simulink model "ex_long_lat_dynamics_charcrit_speed"  (R2026a)
settings: Solver=VariableStepAuto  StopTime=10
libraries: aerolibconvert2 x2, simulink x1
settings Model: Creator=doyeop  LastModifiedBy=doyeop

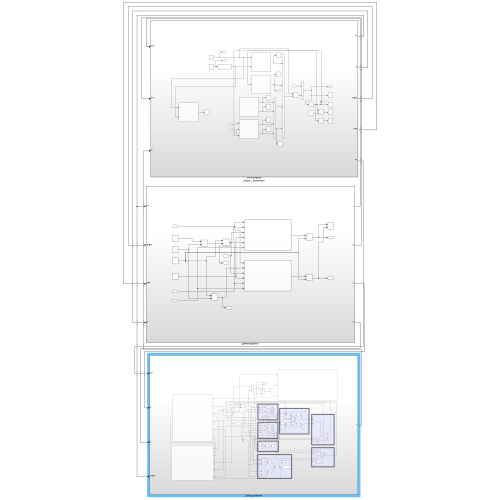
[thumbnail: Simulink's stored preview of the top-level diagram]
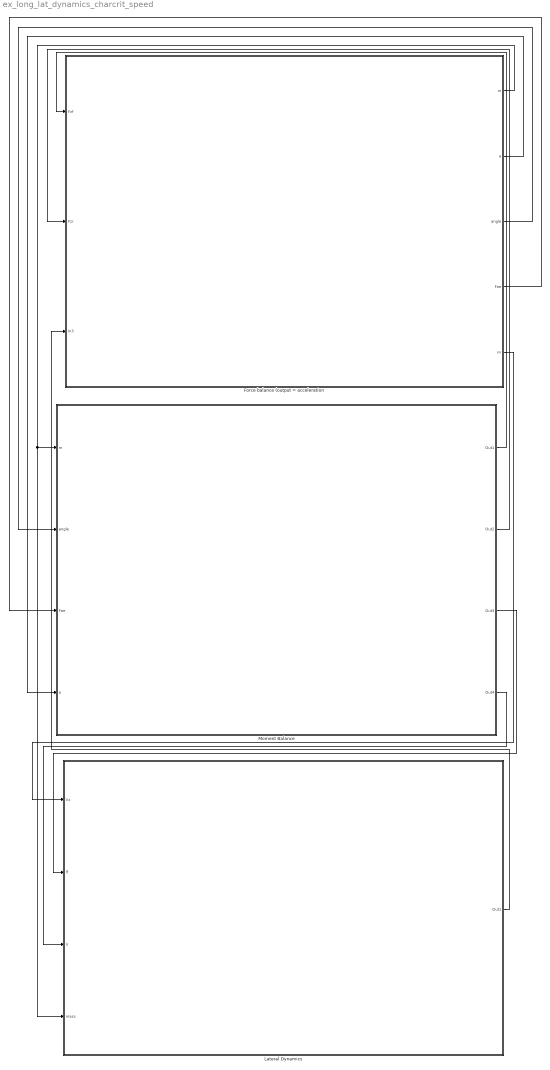
== system ex_long_lat_dynamics_charcrit_speed ==
  Force balance (output = acceleration : Subsystem
  Lateral Dynamics : Subsystem
  Moment Balance : Subsystem
  wires:
  Force balance (output = acceleration/1(m) -> Lateral Dynamics/4(mass), Moment Balance/1(m)
  Force balance (output = acceleration/2(a) -> Moment Balance/4(a)
  Force balance (output = acceleration/3(angle) -> Moment Balance/2(angle)
  Force balance (output = acceleration/4(Fae) -> Moment Balance/3(Fae)
  Moment Balance/1(Out1) -> Force balance (output = acceleration/1(Fzf)
  Moment Balance/2(Out2) -> Force balance (output = acceleration/2(Fzr)
  Force balance (output = acceleration/5(vx) -> Lateral Dynamics/1(Vx)
  Moment Balance/3(Out3) -> Lateral Dynamics/2(lf)
  Moment Balance/4(Out4) -> Lateral Dynamics/3(lr)
  Lateral Dynamics/1(Out1) -> Force balance (output = acceleration/3(In3)

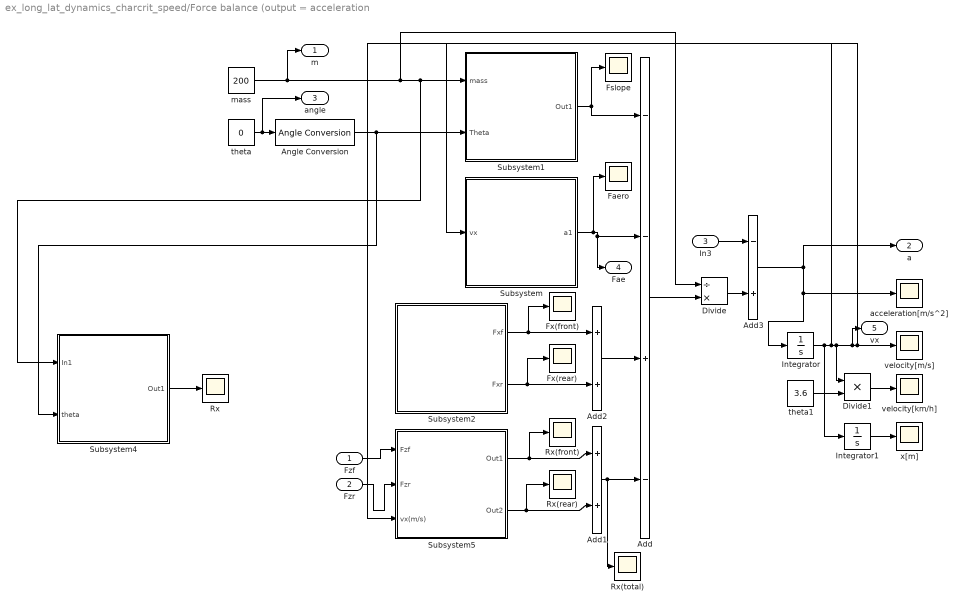
== system ex_long_lat_dynamics_charcrit_speed/Force balance (output = acceleration ==
  Fzf : Inport
  Fzr : Inport  Port=2
  In3 : Inport  Port=3
  Add : Sum  Inputs=--+-
  Add1 : Sum
  Add2 : Sum
  Add3 : Sum  Inputs=-+
  Angle Conversion : aerolibconvert2/Angle Conversion  IU=deg  OU=rad
  Divide : Product  Inputs=/*
  Divide1 : Product  Inputs=**
  Faero : Scope
      settings: ActiveDisplayYMinimum=-21.806973838724872  ActiveDisplayYMaximum=245.93181269445461  DataLoggingVariableName=ScopeData4
  Fslope : Scope
      settings: ActiveDisplayYMinimum=467.68768501992645  ActiveDisplayYMaximum=4126.826484026702  DataLoggingVariableName=ScopeData3
  Fx(front) : Scope
      settings: ActiveDisplayYMinimum=-0.77322383064043154  ActiveDisplayYMaximum=0.91988628090500946  DataLoggingVariableName=ScopeData5
  Fx(rear) : Scope
      settings: ActiveDisplayYMinimum=-0.77322383064043154  ActiveDisplayYMaximum=0.91988628090500946  DataLoggingVariableName=ScopeData10
  Integrator : Integrator
  Integrator1 : Integrator
  Rx : Scope
      settings: ActiveDisplayYMinimum=21.392000000000003  ActiveDisplayYMaximum=41.392  DataLoggingVariableName=ScopeData6
  Rx(front) : Scope
      settings: ActiveDisplayYMinimum=-1  ActiveDisplayYMaximum=1  DataLoggingVariableName=ScopeData11
  Rx(rear) : Scope
      settings: ActiveDisplayYMinimum=-1  ActiveDisplayYMaximum=1  DataLoggingVariableName=ScopeData12
  Rx(total) : Scope
      settings: ActiveDisplayYMinimum=26.459225679325527  ActiveDisplayYMaximum=38.083177364358953  DataLoggingVariableName=ScopeData13
  Subsystem : Subsystem
  Subsystem1 : Subsystem
  Subsystem2 : Subsystem
  Subsystem4 : Subsystem
  Subsystem5 : Subsystem
  acceleration[m/s^2] : Scope
      settings: ActiveDisplayYMinimum=-1  ActiveDisplayYMaximum=1
  mass : Constant  Value=200  SampleTime=-1
  theta : Constant  Value=0  SampleTime=-1
  theta1 : Constant  Value=3.6  SampleTime=-1
  velocity[km/h] : Scope
      settings: ActiveDisplayYMinimum=-12.890564976943338  ActiveDisplayYMaximum=101.85529757372632  DataLoggingVariableName=ScopeData7
  velocity[m/s] : Scope
      settings: ActiveDisplayYMinimum=-1  ActiveDisplayYMaximum=1
  x[m] : Scope
      settings: ActiveDisplayYMinimum=-1  ActiveDisplayYMaximum=1  DataLoggingVariableName=ScopeData2
  m : Outport
  a : Outport  Port=2
  angle : Outport  Port=3
  Fae : Outport  Port=4
  vx : Outport  Port=5
  wires:
  Divide1/1 -> velocity[km/h]/1
  Subsystem/1(a1) -> Faero/1, Add/2, Fae/1
  Integrator1/1 -> x[m]/1
  Add/1 -> Divide/2
  Angle Conversion/1 -> Subsystem4/2(theta), Subsystem1/2(Theta)
  Divide/1 -> Add3/2
  mass/1 -> m/1, Divide/1, Subsystem4/1(In1), Subsystem1/1(mass)
  Subsystem2/1(Fxf) -> Add2/1, Fx(front)/1
  theta1/1 -> Divide1/2
  Integrator/1 -> Integrator1/1, Subsystem/1(vx), Divide1/1, vx/1, Subsystem5/3(vx(m/s)), velocity[m/s]/1
  Subsystem1/1(Out1) -> Fslope/1, Add/1
  Subsystem4/1(Out1) -> Rx/1
  theta/1 -> angle/1, Angle Conversion/1
  Subsystem2/2(Fxr) -> Fx(rear)/1, Add2/2
  Fzf/1 -> Subsystem5/1(Fzf)
  Fzr/1 -> Subsystem5/2(Fzr)
  Add1/1 -> Add/4, Rx(total)/1
  Subsystem5/2(Out2) -> Rx(rear)/1, Add1/2
  Subsystem5/1(Out1) -> Rx(front)/1, Add1/1
  Add2/1 -> Add/3
  In3/1 -> Add3/1
  Add3/1 -> Integrator/1, acceleration[m/s^2]/1, a/1

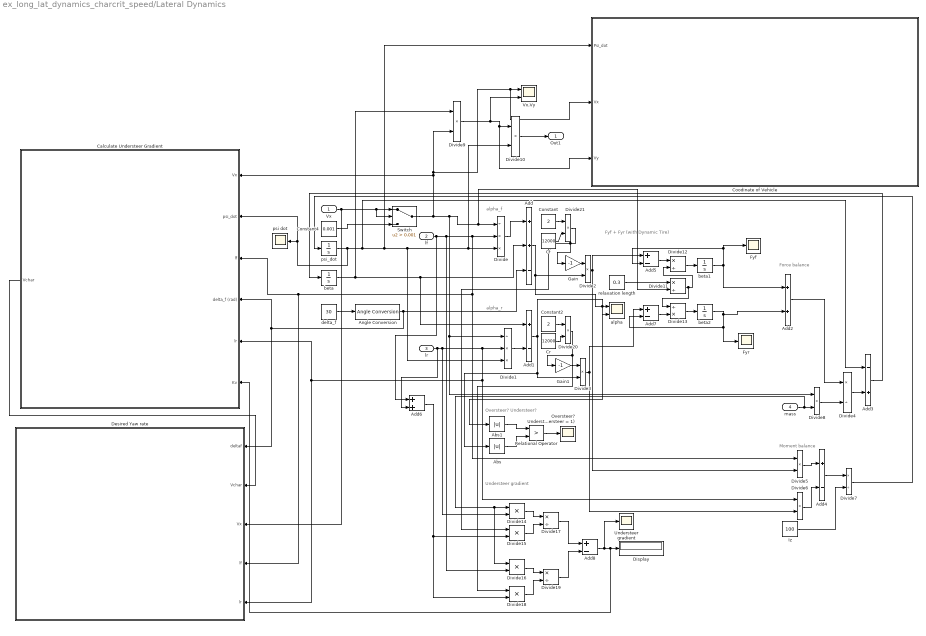
== system ex_long_lat_dynamics_charcrit_speed/Lateral Dynamics ==
  note: Understeer gradient
  note: Oversteer? Understeer?
  note: Moment balance
  note: Force balance
  note: Fyf + Fyr (with Dynamic Tire)
  note: alpha_r
  note: alpha_f
  Vx : Inport
  lf : Inport  Port=2
  lr : Inport  Port=3
  mass : Inport  Port=4
  Abs : Abs  SaturateOnIntegerOverflow=off
  Abs1 : Abs  SaturateOnIntegerOverflow=off
  Add : Sum  Inputs=++-
  Add{1,4..5,7..8} (5 alike) : Sum  Inputs=+-
  Add2 : Sum
  Add3 : Sum  Inputs=-+
  Add6 : Sum
  Angle Conversion : aerolibconvert2/Angle Conversion  IU=deg  OU=rad
  Calculate Understeer Gradient : Subsystem
  Cf : Constant  Value=12000  SampleTime=-1
  Constant : Constant  Value=2  SampleTime=-1
  Constant2 : Constant  Value=2  SampleTime=-1
  Constant4 : Constant  Value=0.001
  Coodinate of Vehicle : Subsystem
  Cr : Constant  Value=12000  SampleTime=-1
  Desired Yaw rate : Subsystem
  Display : Display
  Divide : Product  Inputs=/**
  Divide1 : Product  Inputs=/**
  Divide{5..6,8..10,14..16,18} (9 alike) : Product  Inputs=**
  Divide{4,7,11..12,17,19} (6 alike) : Product  Inputs=*/
  Divide13 : Product  Inputs=/*
  Divide{2..3,20..21} (4 alike) : Product
  Fyf : Scope
      settings: ActiveDisplayYMinimum=-170.39599626491659  ActiveDisplayYMaximum=1134.9817554046469  DataLoggingVariableName=ScopeData14
  Fyr : Scope
      settings: ActiveDisplayYMinimum=-197.89133133597571  ActiveDisplayYMaximum=765.23113635108643  DataLoggingVariableName=ScopeData15
  Gain : Gain  Gain=-1
  Gain1 : Gain  Gain=-1
  Iz : Constant  Value=100  SampleTime=-1
  Oversteer? Understeer? (Understeer = 1) : Scope
      settings: ActiveDisplayYMinimum=-0.12499999999999997  ActiveDisplayYMaximum=1.125  DataLoggingVariableName=ScopeData28
  Relational Operator : RelationalOperator  Operator=>  OutDataTypeStr=boolean  RndMeth=Simplest  InputSameDT=off
  Switch : Switch  Criteria=u2 > Threshold  Threshold=0.001  SaturateOnIntegerOverflow=off  InputSameDT=off
  Understeer gradient : Scope
      settings: ActiveDisplayYMinimum=0.0006666666666666661  ActiveDisplayYMaximum=0.0026666666666666661  DataLoggingVariableName=ScopeData9
  Vx,Vy : Scope  NumInputPorts=2
      settings: ActiveDisplayYMinimum=-0.84716123690803014  ActiveDisplayYMaximum=7.6244511321722737  DataLoggingVariableName=ScopeData16
  alpha : Scope  NumInputPorts=2
      settings: ActiveDisplayYMinimum=-0.10159314992994704  ActiveDisplayYMaximum=0.04167372337235864  DataLoggingVariableName=ScopeData27
  beta : Integrator
  beta1 : Integrator
  beta2 : Integrator
  delta_f : Constant  Value=30  SampleTime=-1
  psi dot : Scope
      settings: ActiveDisplayYMinimum=-0.20399598787459142  ActiveDisplayYMaximum=1.8359638908713232  DataLoggingVariableName=ScopeData17
  psi_dot : Integrator
  relaxation length : Constant  Value=0.3
  Out1 : Outport
  wires:
  beta/1 -> Divide9/1, Add1/1, Add/2
  Divide/1 -> Add/1
  lr/1 -> Add6/2, Divide14/2, Divide6/1, Desired Yaw rate/5(lr), Calculate Understeer Gradient/5(lr), Divide1/2
  Divide1/1 -> Add1/2
  Add/1 -> Abs1/1, alpha/1, Divide2/2
  Cf/1 -> Divide21/2
  Add1/1 -> Abs/1, Divide3/2, alpha/2
  Cr/1 -> Divide20/2
  Divide2/1 -> Add5/1, Divide5/2
  Divide3/1 -> Add7/1, Divide6/2
  Divide4/1 -> Add3/2
  Add3/1 -> beta/1
  lf/1 -> Divide16/2, Divide5/1, Desired Yaw rate/4(lf), Calculate Understeer Gradient/3(lf), Divide/2, Add6/1
  Divide5/1 -> Add4/1
  Divide6/1 -> Add4/2
  Add4/1 -> Divide7/1
  Iz/1 -> Divide7/2
  Divide7/1 -> psi_dot/1
  Vx/1 -> Switch/2, Switch/1, Desired Yaw rate/3(Vx)
  Constant4/1 -> Switch/3
  mass/1 -> Divide14/1, Divide16/1, Divide8/2
  Divide8/1 -> Divide4/2
  Add2/1 -> Divide4/1
  delta_f/1 -> Angle Conversion/1
  beta1/1 -> Fyf/1, Add5/2, Add2/1
  beta2/1 -> Add7/2, Fyr/1, Add2/2
  Abs1/1 -> Relational Operator/1
  Abs/1 -> Relational Operator/2
  Relational Operator/1 -> Oversteer? Understeer? (Understeer = 1)/1
  Divide9/1 -> Coodinate of Vehicle/3(Vy), Divide10/1, Vx,Vy/2
  Divide10/1 -> Out1/1
  Switch/1 -> Divide8/1, Divide1/1, Divide11/2, Divide/1, Divide9/2, Coodinate of Vehicle/2(Vx), Vx,Vy/1, Calculate Understeer Gradient/1(Vx)
  Divide12/1 -> beta1/1
  Add5/1 -> Divide12/1
  Divide11/1 -> Divide13/1, Divide12/2
  Add7/1 -> Divide13/2
  Divide13/1 -> beta2/1
  relaxation length/1 -> Divide11/1
  Add6/1 -> Divide18/2, Divide15/2
  Divide14/1 -> Divide17/1
  Divide15/1 -> Divide17/2
  Divide16/1 -> Divide19/1
  Divide18/1 -> Divide19/2
  Divide19/1 -> Add8/2
  Divide17/1 -> Add8/1
  Add8/1 -> Calculate Understeer Gradient/6(Kv), Display/1, Understeer gradient/1
  Angle Conversion/1 -> Add/3, Desired Yaw rate/1(deltaf), Calculate Understeer Gradient/4(delta_f (rad))
  psi_dot/1 -> psi dot/1, Calculate Understeer Gradient/2(psi_dot), Add3/1, Coodinate of Vehicle/1(Psi_dot), Divide/3, Divide10/2, Divide1/3
  Constant2/1 -> Divide20/1
  Divide20/1 -> Gain1/1, Divide18/1
  Constant/1 -> Divide21/1
  Divide21/1 -> Divide15/1, Gain/1
  Gain/1 -> Divide2/1
  Gain1/1 -> Divide3/1
  Calculate Understeer Gradient/1(Vchar) -> Desired Yaw rate/2(Vchar)

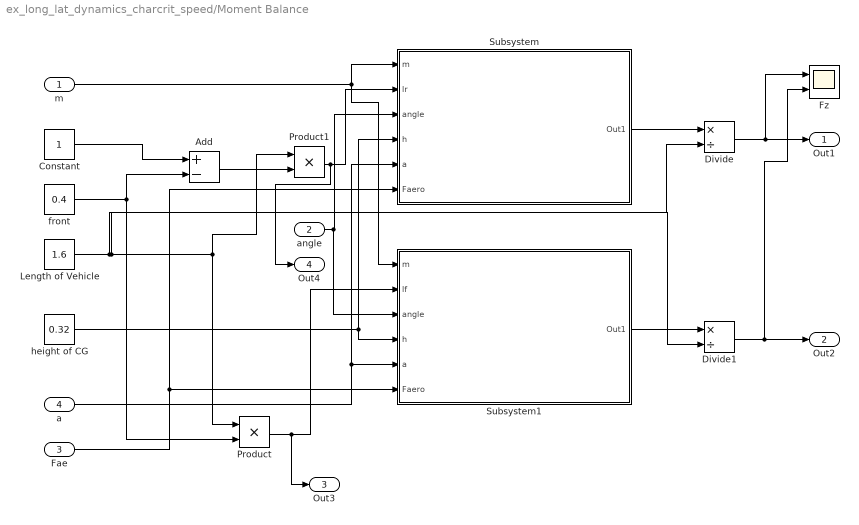
== system ex_long_lat_dynamics_charcrit_speed/Moment Balance ==
  m : Inport
  angle : Inport  Port=2
  Fae : Inport  Port=3
  a : Inport  Port=4
  Add : Sum  Inputs=+-
  Constant : Constant
  Divide : Product  Inputs=*/
  Divide1 : Product  Inputs=*/
  Fz : Scope  NumInputPorts=2
      settings: ActiveDisplayYMinimum=618.58251067683113  ActiveDisplayYMaximum=1343.5454915820123  DataLoggingVariableName=ScopeData8
  Length of Vehicle : Constant  Value=1.6  SampleTime=-1
  Product : Product
  Product1 : Product
  Subsystem : Subsystem
  Subsystem1 : Subsystem
  front : Constant  Value=0.4  SampleTime=-1
  height of CG : Constant  Value=0.32
  Out1 : Outport
  Out2 : Outport  Port=2
  Out3 : Outport  Port=3
  Out4 : Outport  Port=4
  wires:
  m/1 -> Subsystem1/1(m), Subsystem/1(m)
  angle/1 -> Subsystem1/3(angle), Subsystem/3(angle)
  front/1 -> Product/2, Add/2
  Constant/1 -> Add/1
  Length of Vehicle/1 -> Divide/2, Divide1/2, Product1/1, Product/1
  Add/1 -> Product1/2
  Product1/1 -> Out4/1, Subsystem/2(lr)
  height of CG/1 -> Subsystem/4(h), Subsystem1/4(h)
  a/1 -> Subsystem1/5(a), Subsystem/5(a)
  Fae/1 -> Subsystem1/6(Faero), Subsystem/6(Faero)
  Subsystem/1(Out1) -> Divide/1
  Subsystem1/1(Out1) -> Divide1/1
  Product/1 -> Out3/1, Subsystem1/2(lf)
  Divide/1 -> Out1/1, Fz/1
  Divide1/1 -> Fz/2, Out2/1

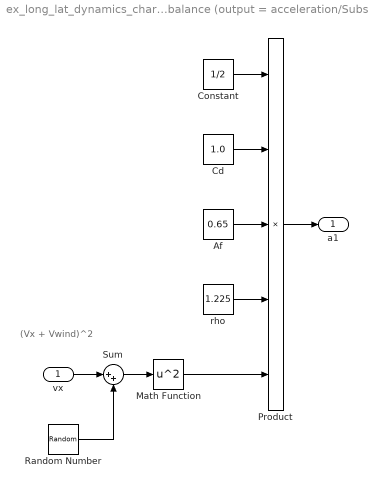
== system ex_long_lat_dynamics_charcrit_speed/Force balance (output = acceleration/Subsystem ==
  note: (Vx + Vwind)^2
  vx : Inport
  Af : Constant  Value=0.65  SampleTime=-1
  Cd : Constant  Value=1.0  SampleTime=-1
  Constant : Constant  Value=1/2  SampleTime=-1
  Math Function : Math  Operator=square
  Product : Product  Inputs=5
  Random Number : RandomNumber  Mean=3  Variance=0.5^2  SampleTime=0.1
  Sum : Sum  Inputs=|++
  rho : Constant  Value=1.225  SampleTime=-1
  a1 : Outport
  wires:
  Cd/1 -> Product/2
  Af/1 -> Product/3
  Constant/1 -> Product/1
  rho/1 -> Product/4
  Random Number/1 -> Sum/2
  vx/1 -> Sum/1
  Sum/1 -> Math Function/1
  Math Function/1 -> Product/5
  Product/1 -> a1/1

== system ex_long_lat_dynamics_charcrit_speed/Force balance (output = acceleration/Subsystem1 ==
  mass : Inport
  Theta : Inport  Port=2
  Constant : Constant  Value=9.81  SampleTime=-1
  Product : Product  Inputs=3
  Trigonometric Function : Trigonometry
  Out1 : Outport
  wires:
  mass/1 -> Product/1
  Theta/1 -> Trigonometric Function/1
  Trigonometric Function/1 -> Product/3
  Constant/1 -> Product/2
  Product/1 -> Out1/1

== system ex_long_lat_dynamics_charcrit_speed/Force balance (output = acceleration/Subsystem2 ==
  Constant : Constant  Value=0  SampleTime=-1
  Constant1 : Constant  Value=500  SampleTime=-1
  Fxf : Outport
  Fxr : Outport  Port=2
  wires:
  Constant/1 -> Fxf/1
  Constant1/1 -> Fxr/1

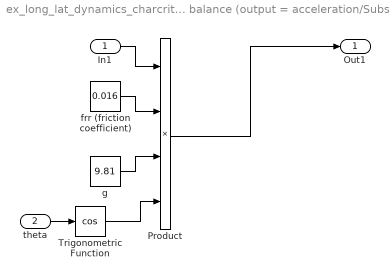
== system ex_long_lat_dynamics_charcrit_speed/Force balance (output = acceleration/Subsystem4 ==
  In1 : Inport
  theta : Inport  Port=2
  Product : Product  Inputs=4
  Trigonometric Function : Trigonometry  Operator=cos
  frr (friction coefficient) : Constant  Value=0.016  SampleTime=-1
  g : Constant  Value=9.81  SampleTime=-1
  Out1 : Outport
  wires:
  In1/1 -> Product/1
  frr (friction coefficient)/1 -> Product/2
  g/1 -> Product/3
  theta/1 -> Trigonometric Function/1
  Product/1 -> Out1/1
  Trigonometric Function/1 -> Product/4

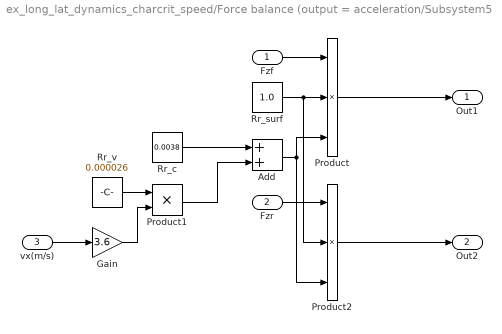
== system ex_long_lat_dynamics_charcrit_speed/Force balance (output = acceleration/Subsystem5 ==
  Fzf : Inport
  Fzr : Inport  Port=2
  vx(m/s) : Inport  Port=3
  Add : Sum
  Gain : Gain  Gain=3.6
  Product : Product  Inputs=3
  Product1 : Product
  Product2 : Product  Inputs=3
  Rr_c : Constant  Value=0.0038  SampleTime=-1
  Rr_surf : Constant  Value=1.0  SampleTime=-1
  Rr_v : Constant  Value=0.000026  SampleTime=-1
  Out1 : Outport
  Out2 : Outport  Port=2
  wires:
  Fzf/1 -> Product/1
  Product/1 -> Out1/1
  Rr_surf/1 -> Product2/2, Product/2
  Rr_v/1 -> Product1/1
  vx(m/s)/1 -> Gain/1
  Product1/1 -> Add/2
  Rr_c/1 -> Add/1
  Add/1 -> Product2/3, Product/3
  Gain/1 -> Product1/2
  Fzr/1 -> Product2/1
  Product2/1 -> Out2/1

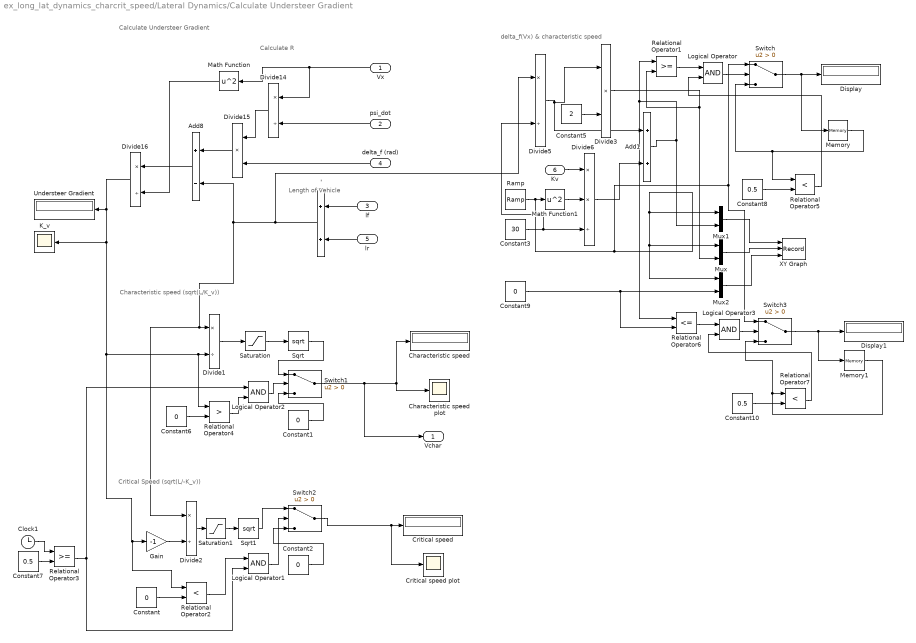
== system ex_long_lat_dynamics_charcrit_speed/Lateral Dynamics/Calculate Understeer Gradient ==
  note: delta_f(Vx) & characteristic speed
  note: Critical Speed
      | (sqrt(L/-K_v))
  note: Characteristic speed
      | (sqrt(L/K_v))
  note: Length of Vehicle
  note: Calculate Understeer Gradient
  note: Calculate R
  Vx : Inport
  psi_dot : Inport  Port=2
  lf : Inport  Port=3
  delta_f (rad) : Inport  Port=4
  lr : Inport  Port=5
  Kv : Inport  Port=6
  ' : Sum
  Add1 : Sum
  Add8 : Sum  Inputs=+-
  Characteristic speed : Display
  Characteristic speed plot : Scope
      settings: ActiveDisplayYMinimum=-3.8779477371123048  ActiveDisplayYMaximum=34.90152963401075  DataLoggingVariableName=ScopeData19
  Clock1 : Clock
  Constant{,1..2,6} (4 alike) : Constant  Value=0
  Constant10 : Constant  Value=0.5
  Constant3 : Constant  Value=30
  Constant5 : Constant  Value=2
  Constant7 : Constant  Value=0.5  SampleTime=-1
  Constant8 : Constant  Value=0.5
  Constant9 : Constant  Value=0  SampleTime=-1
  Critical speed : Display
  Critical speed plot : Scope
      settings: ActiveDisplayYMinimum=-4.4232312925042283  ActiveDisplayYMaximum=39.80908163253806  DataLoggingVariableName=ScopeData21
  Display : Display
  Display1 : Display
  Divide{1..2,5,14,16} (5 alike) : Product  Inputs=*/
  Divide15 : Product  Inputs=**
  Divide3 : Product  Inputs=**
  Divide6 : Product  Inputs=**/
  Gain : Gain  Gain=-1
  K_v : Scope
      settings: ActiveDisplayYMinimum=-33.664212716268274  ActiveDisplayYMaximum=291.42077077577937  DataLoggingVariableName=ScopeData18
  Logical Operator{,1..3} (4 alike) : Logic  AllPortsSameDT=off  OutDataTypeStr=boolean
  Math Function : Math  Operator=square
  Math Function1 : Math  Operator=square
  Memory : Memory
  Memory1 : Memory
  Mux : Mux  Inputs=2
  Mux1 : Mux  Inputs=2
  Mux2 : Mux  Inputs=2
  Ramp : simulink/Sources/Ramp  slope=10  start=0  InitialOutput=0
  Relational Operator1 : RelationalOperator  OutDataTypeStr=boolean  RndMeth=Simplest  InputSameDT=off
  Relational Operator2 : RelationalOperator  Operator=<  OutDataTypeStr=boolean  RndMeth=Simplest  InputSameDT=off
  Relational Operator3 : RelationalOperator  OutDataTypeStr=boolean  RndMeth=Simplest  InputSameDT=off
  Relational Operator4 : RelationalOperator  Operator=>  OutDataTypeStr=boolean  RndMeth=Simplest  InputSameDT=off
  Relational Operator5 : RelationalOperator  Operator=<  OutDataTypeStr=boolean  RndMeth=Simplest  InputSameDT=off
  Relational Operator6 : RelationalOperator  Operator=<=  OutDataTypeStr=boolean  RndMeth=Simplest  InputSameDT=off
  Relational Operator7 : RelationalOperator  Operator=<  OutDataTypeStr=boolean  RndMeth=Simplest  InputSameDT=off
  Saturation : Saturate  UpperLimit=inf  LowerLimit=0
  Saturation1 : Saturate  UpperLimit=inf  LowerLimit=0
  Sqrt : Sqrt
  Sqrt1 : Sqrt
  Switch{,1..3} (4 alike) : Switch  Criteria=u2 > Threshold  SaturateOnIntegerOverflow=off  InputSameDT=off
  Understeer Gradient : Display
  XY Graph : Record  NumPorts=3.0  FileSettingsInternal="{\"entries\":[{\"content\":{\"excelSettings\":{\"content\":{},\"type\":\"Streamout.ExcelSettings\"},\"parquetSettings\":{\"content\":{},\"type\":\"Streamout.ParquetSettings\"}},\"type\":\"Streamout.FileSettingStorage\",\"uuid\":\"\"}],\"packageUris\":[\"http:\\/\\/schema.mathworks.com\\/mf0\\/streamout_blocks\\/R2020a\"],\"version\":\"1.0\"}"  FrameSettings=[0, 0, 0]  Layout=[1 1]  SignalsInternal="{\"entries\":[{\"content\":{\"signals\":[{\"content\":{\"blockPath\":[],\"dimensions\":[2],\"domain\":\"\",\"hasChildren\":true,\"lineColor\":\"#22b573\",\"lineWidth\":2,\"port\":1,\"sid\":[\"\"],\"signalID\":1,\"signalName\":\"Mux1\"},\"type\":\"RecordBlkView.Signal\",\"uuid\":\"\"},{\"content\":{\"blockPath\":[],\"channel\":[1],\"dimensions\":[2],\"domain\":\"\",\"lineColor\":\"#64d413\",\"lineWidth\":2,\"parentID\":1,\"plots\":[ 1 ],\"port\":1,\"sid\":[\"\"],\"signalID\":2,\"signalName\":\"Mux1\"},\"type\":\"RecordBlkView.Signal\",\"uuid\":\"\"},{\"content\":{\"blockPath\":[],\"dimensions\":[2],\"domain\":\"\",\"hasChildren\":true,\"lineColor\":\"#d95319\",\"lineWidth\":2,\"port\":2,\"sid\":[\"\"],\"signalID\":3,\"signalName\":\"Mux\"},\"type\":\"RecordBlkView.Signal\",\"uuid\":\"\"},{\"content\":{\"blockPath\":[],\"channel\":[1],\"dimensions\":[2],\"domain\":\"\",\"lineColor\":\"#22b573\",\"lineWidth\":2,\"parentID\":3,\"plots\":[ 1 ],\"port\":2,\"sid\":[\"\"],\"signalID\":4,\"signalName\":\"Mux\"},\"type\":\"RecordBlkView.Signal\",\"uuid\":\"\"},{\"content\":{\"blockPath\":[],\"dimensions\":[2],\"domain\":\"\",\"hasChildren\":true,\"lineColor\":\"#7e2f8e\",\"lineWidth\":2,\"port\":3,\"sid\":[\"\"],\"signalID\":5,\"signalName\":\"Mux2\"},\"type\":\"RecordBlkView.Signal\",\"uuid\":\"\"},{\"content\":{\"blockPath\":[],\"channel\":[1],\"dimensions\":[2],\"domain\":\"\",\"lineColor\":\"#ff6929\",\"lineWidth\":2,\"parentID\":5,\"plots\":[ 1 ],\"port\":3,\"sid\":[\"\"],\"signalID\":6,\"signalName\":\"Mux2\"},\"type\":\"RecordBlkView.Signal\",\"uuid\":\"\"},{\"content\":{\"blockPath\":[],\"channel\":[2],\"dimensions\":[2],\"domain\":\"\",\"lineColor\":\"#d95319\",\"lineWidth\":2,\"parentID\":1,\"plots\":[ 1 ],\"port\":1,\"sid\":[\"\"],\"signalID\":7,\"signalName\":\"Mux1\"},\"type\":\"RecordBlkView.Signal\",\"uuid\":\"\"},{\"content\":{\"blockPath\":[],\"channel\":[2],\"dimensions\":[2],\"domain\":\"\",\"lineColor\":\"#edb120\",\"lineWidth\":2,\"parentID\":3,\"plots\":[ 1 ],\"port\":2,\"sid\":[\"\"],\"signalID\":8,\"signalName\":\"Mux\"},\"type\":\"RecordBlkView.Signal\",\"uuid\":\"\"},{\"content\":{\"blockPath\":[],\"channel\":[2],\"dimensions\":[2],\"domain\":\"\",\"lineColor\":\"#22b573\",\"lineWidth\":2,\"parentID\":5,\"plots\":[ 1 ],\"port\":3,\"sid\":[\"\"],\"signalID\":9,\"signalName\":\"Mux2\"},\"type\":\"RecordBlkView.Signal\",\"uuid\":\"\"}]},\"type\":\"RecordBlkView.InputSignals\",\"uuid\":\"\"}],\"packageUris\":[\"http:\\/\\/schema.mathworks.com\\/mf0\\/streamout_blocks\\/R2020a\"],\"version\":\"1.0\"}"  VisualizationBindings="{\"xyplotplugin\":{\"info\":[{\"series\":[{\"bindingParametersList\":[{\"parameter\":\"X-Axis\",\"signalID\":2,\"signalName\":\"Mux1(1)\"},{\"parameter\":\"Y-Axis\",\"signalID\":7,\"signalName\":\"Mux1(2)\"},{\"parameter\":\"X-Axis\",\"signalID\":2,\"signalName\":\"Mux1(1)\"},{\"parameter\":\"Y-Axis\",\"signalID\":7,\"signalName\":\"Mux1(2)\"},{\"parameter\":\"X-Axis\",\"signalID\":2,\"signalName\":\"Mux1(1)\"},{\"parameter\":\"Y-Axis\",\"signalID\":7,\"signalName\":\"Mux1(2)\"}],\"seriesID\":0},{\"bindingParametersList\":[{\"parameter\":\"X-Axis\",\"signalID\":4,\"signalName\":\"Mux(1)\"},{\"parameter\":\"Y-Axis\",\"signalID\":8,\"signalName\":\"Mux(2)\"},{\"parameter\":\"X-Axis\",\"signalID\":4,\"signalName\":\"Mux(1)\"},{\"parameter\":\"Y-Axis\",\"signalID\":8,\"signalName\":\"Mux(2)\"},{\"parameter\":\"X-Axis\",\"signalID\":4,\"signalName\":\"Mux(1)\"},{\"parameter\":\"Y-Axis\",\"signalID\":8,\"signalName\":\"Mux(2)\"}],\"seriesID\":1},{\"bindingParametersList\":[{\"parameter\":\"X-Axis\",\"signalID\":6,\"signalName\":\"Mux2(1)\"},{\"parameter\":\"Y-Axis\",\"signalID\":9,\"signalName\":\"Mux2(2)\"}],\"seriesID\":2}],\"subplotID\":1}]}}"  CompatibilityTag=XY
  Vchar : Outport
  wires:
  lr/1 -> '/2
  delta_f (rad)/1 -> Divide15/2
  Add8/1 -> Divide16/1
  Math Function/1 -> Divide16/2
  lf/1 -> '/1
  Divide15/1 -> Add8/1
  psi_dot/1 -> Divide14/2
  Divide1/1 -> Saturation/1
  Constant1/1 -> Switch1/3
  Saturation/1 -> Sqrt/1
  Divide2/1 -> Saturation1/1
  Saturation1/1 -> Sqrt1/1
  Sqrt/1 -> Switch1/1
  Switch2/1 -> Critical speed plot/1, Critical speed/1
  Vx/1 -> Divide14/1, Math Function/1
  Relational Operator3/1 -> Logical Operator2/1, Logical Operator1/2
  Clock1/1 -> Relational Operator3/1
  Constant7/1 -> Relational Operator3/2
  Divide16/1 -> Relational Operator2/1, Gain/1, Relational Operator4/1, Divide1/2, K_v/1, Understeer Gradient/1
  Switch1/1 -> Vchar/1, Characteristic speed plot/1, Characteristic speed/1
  Logical Operator2/1 -> Switch1/2
  Logical Operator1/1 -> Switch2/2
  Constant/1 -> Relational Operator2/2
  Relational Operator2/1 -> Logical Operator1/1
  Constant2/1 -> Switch2/3
  Sqrt1/1 -> Switch2/1
  Constant6/1 -> Relational Operator4/2
  Relational Operator4/1 -> Logical Operator2/2
  Divide14/1 -> Divide15/1
  Divide6/1 -> Add1/2
  Divide5/1 -> Divide3/1, Add1/1
  Math Function1/1 -> Divide6/2
  Constant3/1 -> Divide5/2, Divide6/3
  Kv/1 -> Divide6/1
  Constant5/1 -> Divide3/2
  Divide3/1 -> Mux/2, Relational Operator1/2
  Add1/1 -> Mux1/2, Relational Operator1/1, Relational Operator6/1
  Mux/1 -> XY Graph/2
  Mux1/1 -> XY Graph/1
  Relational Operator1/1 -> Logical Operator/1
  Relational Operator5/1 -> Logical Operator/2
  Memory/1 -> Switch/3, Relational Operator5/1
  Logical Operator/1 -> Switch/2
  Switch/1 -> Memory/1, Display/1
  Ramp/1 -> Mux1/1, Mux2/1, Mux/1, Switch/1, Switch3/1, Math Function1/1
  Constant8/1 -> Relational Operator5/2
  Gain/1 -> Divide2/2
  '/1 -> Divide5/1, Divide2/1, Divide1/1, Add8/2
  Constant9/1 -> Relational Operator6/2, Mux2/2
  Mux2/1 -> XY Graph/3
  Relational Operator6/1 -> Logical Operator3/1
  Logical Operator3/1 -> Switch3/2
  Switch3/1 -> Display1/1, Memory1/1
  Memory1/1 -> Switch3/3, Relational Operator7/1
  Relational Operator7/1 -> Logical Operator3/2
  Constant10/1 -> Relational Operator7/2

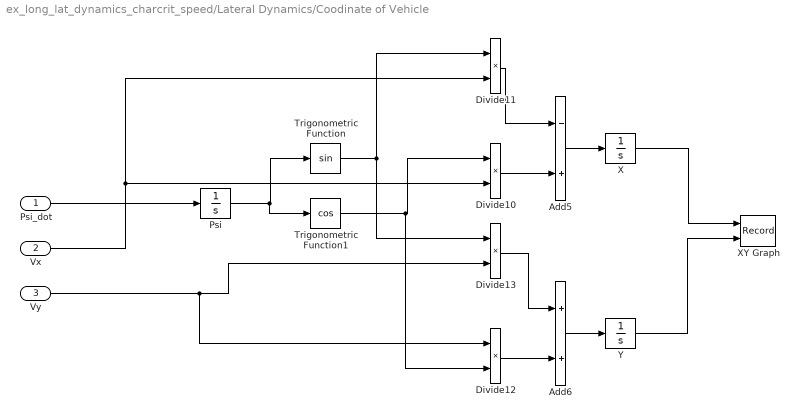
== system ex_long_lat_dynamics_charcrit_speed/Lateral Dynamics/Coodinate of Vehicle ==
  Psi_dot : Inport
  Vx : Inport  Port=2
  Vy : Inport  Port=3
  Add5 : Sum  Inputs=-+
  Add6 : Sum
  Divide{10..13} (4 alike) : Product  Inputs=**
  Psi : Integrator
  Trigonometric Function : Trigonometry
  Trigonometric Function1 : Trigonometry  Operator=cos
  X : Integrator
  XY Graph : Record  NumPorts=2.0  FileSettingsInternal="{\"entries\":[{\"content\":{\"excelSettings\":{\"content\":{},\"type\":\"Streamout.ExcelSettings\"},\"parquetSettings\":{\"content\":{},\"type\":\"Streamout.ParquetSettings\"}},\"type\":\"Streamout.FileSettingStorage\",\"uuid\":\"\"}],\"packageUris\":[\"http:\\/\\/schema.mathworks.com\\/mf0\\/streamout_blocks\\/R2020a\"],\"version\":\"1.0\"}"  FrameSettings=[0, 0]  Layout=[1 1]  SignalsInternal="{\"entries\":[{\"content\":{\"signals\":[{\"content\":{\"blockPath\":[],\"dimensions\":[1],\"domain\":\"\",\"lineColor\":\"#a2142f\",\"plots\":[ 1 ],\"port\":1,\"sid\":[\"\"],\"signalID\":1,\"signalName\":\"X\"},\"type\":\"RecordBlkView.Signal\",\"uuid\":\"\"},{\"content\":{\"blockPath\":[],\"dimensions\":[1],\"domain\":\"\",\"lineColor\":\"#139fff\",\"plots\":[ 1 ],\"port\":2,\"sid\":[\"\"],\"signalID\":2,\"signalName\":\"Y\"},\"type\":\"RecordBlkView.Signal\",\"uuid\":\"\"}]},\"type\":\"RecordBlkView.InputSignals\",\"uuid\":\"\"}],\"packageUris\":[\"http:\\/\\/schema.mathworks.com\\/mf0\\/streamout_blocks\\/R2020a\"],\"version\":\"1.0\"}"  VisualizationBindings="{\"xyplotplugin\":{\"info\":[{\"series\":[{\"bindingParametersList\":[{\"parameter\":\"X-Axis\",\"signalID\":1,\"signalName\":\"X\"},{\"parameter\":\"Y-Axis\",\"signalID\":2,\"signalName\":\"Y\"}],\"seriesID\":0}],\"subplotID\":1}]}}"  CompatibilityTag=XY
  Y : Integrator
  wires:
  X/1 -> XY Graph/1
  Add6/1 -> Y/1
  Divide10/1 -> Add5/2
  Psi/1 -> Trigonometric Function1/1, Trigonometric Function/1
  Divide12/1 -> Add6/2
  Trigonometric Function1/1 -> Divide12/2, Divide10/1
  Y/1 -> XY Graph/2
  Divide13/1 -> Add6/1
  Psi_dot/1 -> Psi/1
  Add5/1 -> X/1
  Trigonometric Function/1 -> Divide11/1, Divide13/1
  Divide11/1 -> Add5/1
  Vx/1 -> Divide11/2, Divide10/2
  Vy/1 -> Divide12/1, Divide13/2

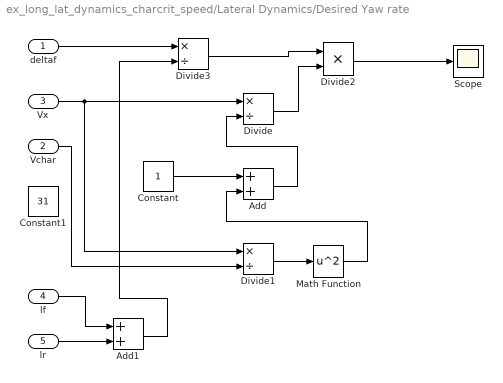
== system ex_long_lat_dynamics_charcrit_speed/Lateral Dynamics/Desired Yaw rate ==
  deltaf : Inport
  Vchar : Inport  Port=2
  Vx : Inport  Port=3
  lf : Inport  Port=4
  lr : Inport  Port=5
  Add : Sum
  Add1 : Sum
  Constant : Constant
  Constant1 : Constant  Value=31
  Divide : Product  Inputs=*/
  Divide1 : Product  Inputs=*/
  Divide2 : Product  Inputs=**
  Divide3 : Product  Inputs=*/
  Math Function : Math  Operator=square
  Scope : Scope
      settings: ActiveDisplayYMinimum=-0.204007327843998  ActiveDisplayYMaximum=1.8360659505959824  DataLoggingVariableName=ScopeData20
  wires:
  Vx/1 -> Divide1/1, Divide/1
  Constant/1 -> Add/1
  Divide1/1 -> Math Function/1
  Math Function/1 -> Add/2
  Add/1 -> Divide/2
  lf/1 -> Add1/1
  lr/1 -> Add1/2
  Divide/1 -> Divide2/2
  deltaf/1 -> Divide3/1
  Add1/1 -> Divide3/2
  Divide3/1 -> Divide2/1
  Divide2/1 -> Scope/1
  Vchar/1 -> Divide1/2

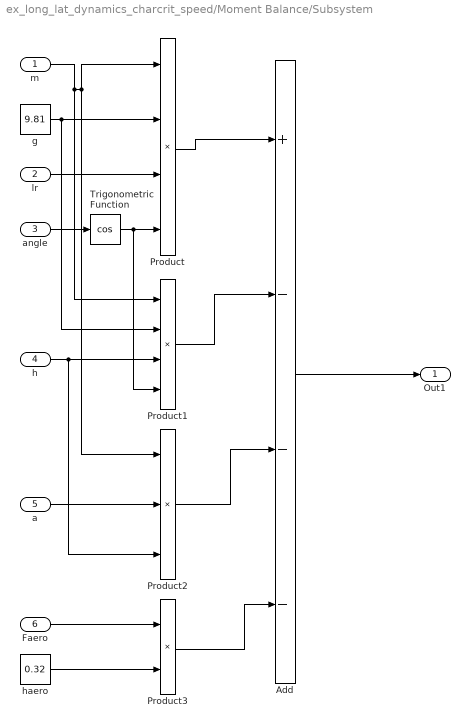
== system ex_long_lat_dynamics_charcrit_speed/Moment Balance/Subsystem ==
  m : Inport
  lr : Inport  Port=2
  angle : Inport  Port=3
  h : Inport  Port=4
  a : Inport  Port=5
  Faero : Inport  Port=6
  Add : Sum  Inputs=+---
  Product : Product  Inputs=4
  Product1 : Product  Inputs=4
  Product2 : Product  Inputs=3
  Product3 : Product
  Trigonometric Function : Trigonometry  Operator=cos
  g : Constant  Value=9.81  SampleTime=-1
  haero : Constant  Value=0.32  SampleTime=-1
  Out1 : Outport
  wires:
  m/1 -> Product1/1, Product2/1, Product/1
  angle/1 -> Trigonometric Function/1
  g/1 -> Product1/2, Product/2
  lr/1 -> Product/3
  Trigonometric Function/1 -> Product1/4, Product/4
  a/1 -> Product2/2
  h/1 -> Product2/3, Product1/3
  haero/1 -> Product3/2
  Faero/1 -> Product3/1
  Product/1 -> Add/1
  Product1/1 -> Add/2
  Product2/1 -> Add/3
  Product3/1 -> Add/4
  Add/1 -> Out1/1

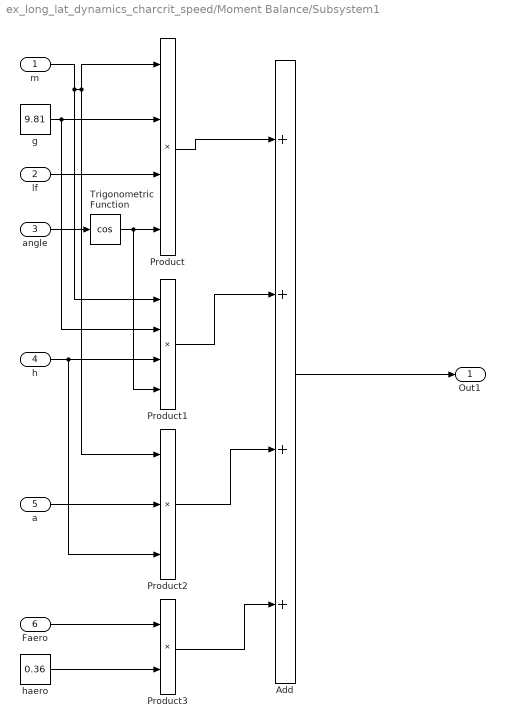
== system ex_long_lat_dynamics_charcrit_speed/Moment Balance/Subsystem1 ==
  m : Inport
  lf : Inport  Port=2
  angle : Inport  Port=3
  h : Inport  Port=4
  a : Inport  Port=5
  Faero : Inport  Port=6
  Add : Sum  Inputs=++++
  Product : Product  Inputs=4
  Product1 : Product  Inputs=4
  Product2 : Product  Inputs=3
  Product3 : Product
  Trigonometric Function : Trigonometry  Operator=cos
  g : Constant  Value=9.81  SampleTime=-1
  haero : Constant  Value=0.36  SampleTime=-1
  Out1 : Outport
  wires:
  m/1 -> Product1/1, Product2/1, Product/1
  angle/1 -> Trigonometric Function/1
  g/1 -> Product1/2, Product/2
  lf/1 -> Product/3
  Trigonometric Function/1 -> Product1/4, Product/4
  a/1 -> Product2/2
  h/1 -> Product2/3, Product1/3
  haero/1 -> Product3/2
  Faero/1 -> Product3/1
  Product/1 -> Add/1
  Product1/1 -> Add/2
  Product2/1 -> Add/3
  Product3/1 -> Add/4
  Add/1 -> Out1/1
